simulink model "Simulink_VDP_comparison"  (R2022a)
settings: Solver=FixedStepAuto  StartTime=0.0  StopTime=Tf  FixedStep=Ts  RelTol=1e-3
values from neighbouring files (symbols this model uses):
  C = zeros(size(Z,1),size(A,2))    [VanDerPol_MPC_Koopman.m]
  D = zeros(size(Z,1),size(U,1))    [VanDerPol_MPC_Koopman.m]
  ss_0 = Spline_Radial_Obs(y_0,X0)    [VanDerPol_MPC_Evaluation.m]
  Ts = 1e-2    (= 0.01)    [VanDerPol_MPC.m]
undefined symbols (not defined in the file or in its folder): A, B
libraries: mpclib x1
settings Model: Creator=sergiovaneg  LastModifiedBy=sergiovaneg

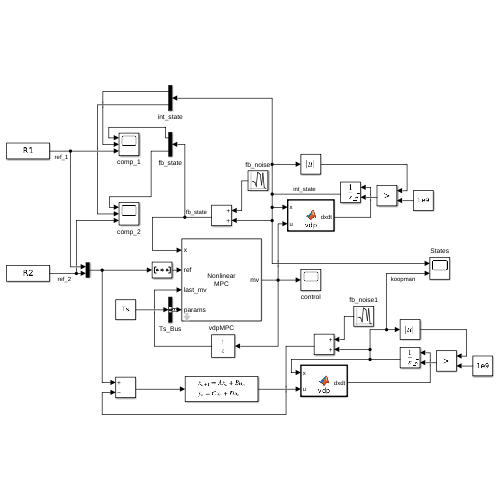
[thumbnail: Simulink's stored preview of the top-level diagram]
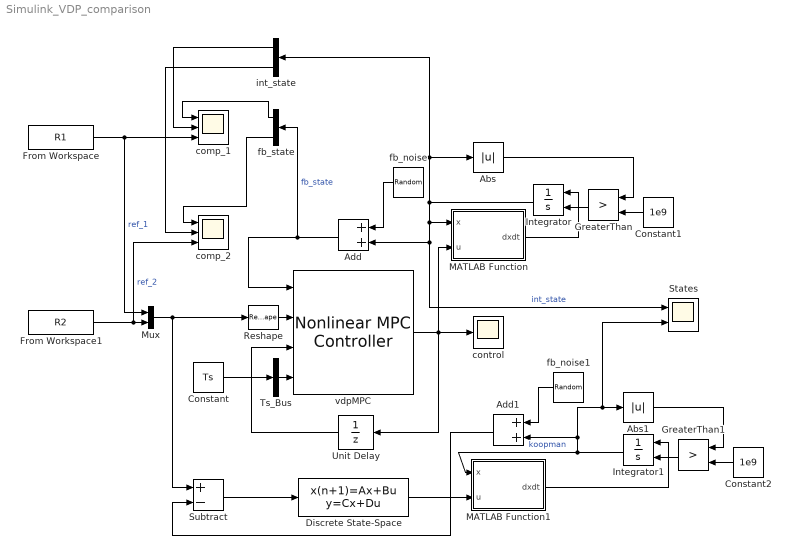
== system Simulink_VDP_comparison ==
  Abs : Abs  SaturateOnIntegerOverflow=off
  Abs1 : Abs  SaturateOnIntegerOverflow=off
  Add : Sum
  Add1 : Sum
  Constant : Constant  Value=Ts
  Constant1 : Constant  Value=1e9  SampleTime=Ts
  Constant2 : Constant  Value=1e9  SampleTime=Ts
  Discrete State-Space : DiscreteStateSpace  A=A  B=B  C=C  D=D  InitialCondition=ss_0  SampleTime=Ts
  From Workspace : FromWorkspace  VariableName=R1
  From Workspace1 : FromWorkspace  VariableName=R2
  GreaterThan : RelationalOperator  Operator=>  OutDataTypeStr=boolean  RndMeth=Simplest  InputSameDT=off
  GreaterThan1 : RelationalOperator  Operator=>  OutDataTypeStr=boolean  RndMeth=Simplest  InputSameDT=off
  Integrator : Integrator  ExternalReset=rising  InitialCondition=[0;0]
  Integrator1 : Integrator  ExternalReset=rising  InitialCondition=[0;0]
  MATLAB Function : MATLAB Function  TreatAsAtomicUnit=on
  MATLAB Function1 : MATLAB Function  TreatAsAtomicUnit=on
  Mux : Mux  Inputs=2
  Reshape : Reshape  OutputDimensionality=Row vector (2-D)
  States : Scope  NumInputPorts=2
  Subtract : Sum  Inputs=+-
  Ts_Bus : BusCreator  Inputs=1  OutDataTypeStr=Bus: Ts_Bus  NonVirtualBus=on
      settings: InheritFromInputs=off
  Unit Delay : UnitDelay  SampleTime=-1  HasFrameUpgradeWarning=on
  comp_1 : Scope  NumInputPorts=3
  comp_2 : Scope  NumInputPorts=3
  control : Scope
  fb_noise : RandomNumber  Variance=0.001  Seed=[2;3]  SampleTime=Ts
  fb_noise1 : RandomNumber  Variance=0.001  Seed=[2;3]  SampleTime=Ts
  fb_state : Demux  Outputs=2
  int_state : Demux  Outputs=2
  vdpMPC : mpclib/Nonlinear MPC Controller  nlmpcobj=nlobj  UseObjectTs=on  UseMEX=off  md_enabled=off  mvtarget_enabled=off  param_enabled=on  cost_enabled=off  mvseq_enabled=off  stateseq_enabled=off  ovseq_enabled=off  slack_enabled=off  status_enabled=off  ov_min=off  ov_max=off  mv_min=off  mv_max=off  mvrate_min=off  mvrate_max=off  state_min=off  state_max=off  ov_weight=off  mv_weight=off  mvrate_weight=off  ecr_weight=off  nlp_initialize=off
  wires:
  Add/1 -> fb_state/1, vdpMPC/1  "fb_state"
  From Workspace/1 -> Mux/1, comp_1/3  "ref_1"
  int_state/1 -> comp_1/2
  fb_noise/1 -> Add/1
  Reshape/1 -> vdpMPC/2
  Abs/1 -> GreaterThan/1
  vdpMPC/1 -> MATLAB Function/2(u), Unit Delay/1, control/1
  Constant/1 -> Ts_Bus/1
  Integrator/1 -> int_state/1, Abs/1, States/1, Add/2, MATLAB Function/1(x)  "int_state"
  GreaterThan/1 -> Integrator/2
  From Workspace1/1 -> comp_2/3, Mux/2  "ref_2"
  Unit Delay/1 -> vdpMPC/3
  int_state/2 -> comp_2/2
  MATLAB Function/1(dxdt) -> Integrator/1
  Mux/1 -> Subtract/1, Reshape/1
  Constant1/1 -> GreaterThan/2
  fb_state/1 -> comp_1/1
  Ts_Bus/1 -> vdpMPC/4
  fb_state/2 -> comp_2/1
  Discrete State-Space/1 -> MATLAB Function1/2(u)
  Abs1/1 -> GreaterThan1/1
  GreaterThan1/1 -> Integrator1/2
  MATLAB Function1/1(dxdt) -> Integrator1/1
  Integrator1/1 -> MATLAB Function1/1(x), Add1/2, States/2, Abs1/1  "koopman"
  Constant2/1 -> GreaterThan1/2
  Subtract/1 -> Discrete State-Space/1
  fb_noise1/1 -> Add1/1
  Add1/1 -> Subtract/2

== matlab function Simulink_VDP_comparison/MATLAB Function ==
  data: x input; u input; dxdt output
function dxdt = vdp(x,u)
    dxdt = zeros(2,1);
    dxdt(1) = 2*x(2);
    dxdt(2) = -0.8*x(1)+2*x(2)-10*(x(1)^2)*x(2)+u;

== matlab function Simulink_VDP_comparison/MATLAB Function1 ==
  data: x input; u input; dxdt output
function dxdt = vdp(x,u)
    dxdt = zeros(2,1);
    dxdt(1) = 2*x(2);
    dxdt(2) = -0.8*x(1)+2*x(2)-10*(x(1)^2)*x(2)+u;
